simulink model "A2_NDI_AttitudeDynamics"  (R2017b)
settings: Solver=VariableStepAuto  StartTime=0.0  StopTime=300  FixedStep=1  MaxStep=0.1  RelTol=1e-6  EnableMultiTasking=on
StopFcn:
  | attitudePlot = animateAttitude(rotmOut, 0.016);
  | attitudePlot.plotInit;
values from neighbouring files (symbols this model uses):
  J_sat = [2.5 2.5 2.5]    [AttitudeDynamicsData.m]
  T_disturb = ones(1,3) * 0.1E-3    [AttitudeDynamicsData.m]
libraries: SatelliteLibrary x11, simulink x1
settings Model: Creator=Huib  LastModifiedBy=Huib
settings DataIOCC: LimitDataPoints=on
settings OptimizationCC: LifeSpan=inf
settings DebuggingCC: AllowSymbolicDim=off  SFUnexpectedBacktrackingDiag=warning  SFNoUnconditionalDefaultTransitionDiag=warning  SFExecutionAtInitializationDiag=none
settings ModelReferenceCC: PropagateSignalLabelsOutOfModel=off
settings CodeAppCC: StateflowObjectComments=on
settings GRTTargetCC: TargetLangStandard=C89/C90 (ANSI)
settings ConfigComp: CovMetricSettings=dw  CovHtmlReporting=on  CovSaveCumulativeToWorkspaceVar=on  CovSaveSingleToWorkspaceVar=on  CovExternalEMLEnable=off

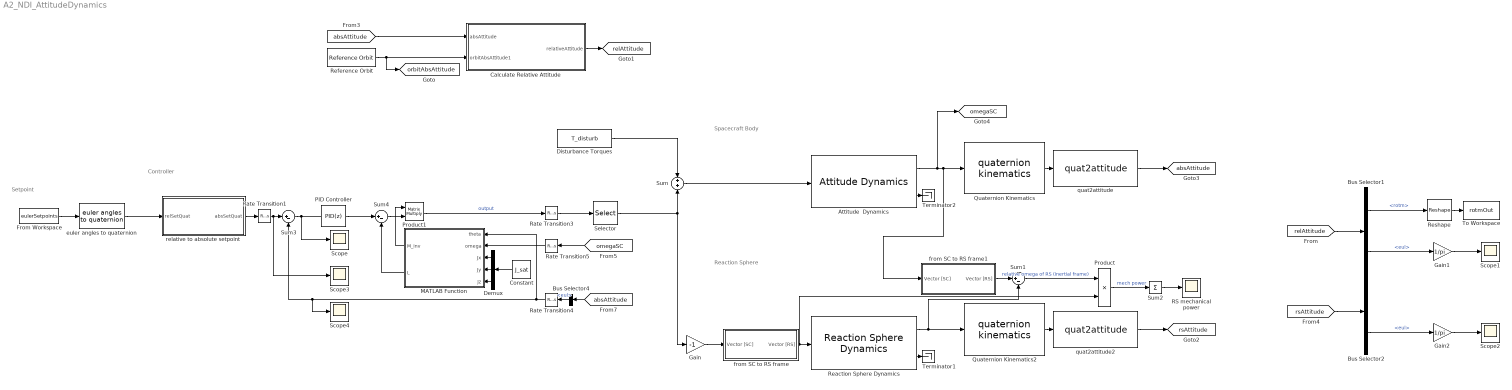
== system A2_NDI_AttitudeDynamics ==
  note: Setpoint
  note: Reaction Sphere
  note: Controller
  note: Spacecraft Body
  Attitude  Dynamics : SatelliteLibrary/Attitude Dynamics  J11=J_sat(1)  J22=J_sat(2)  J33=J_sat(3)  omega0=w_zero
  Bus Selector1 : BusSelector  OutputSignals=rotm,eul
  Bus Selector2 : BusSelector  OutputSignals=rotm,eul
  Bus Selector4 : BusSelector  OutputSignals=eul
  Calculate Relative Attitude : Subsystem
  Constant : Constant  Value=J_sat
  Demux : Demux  Outputs=3
  Disturbance Torques : Constant  Value=T_disturb
  From Workspace : FromWorkspace  VariableName=eulerSetpoints  SampleTime=0  Interpolate=off  OutputAfterFinalValue=Holding final value
  Gain : Gain  Gain=-1
  Gain1 : Gain  Gain=1/pi
  Gain2 : Gain  Gain=1/pi
  MATLAB Function : MATLAB Function  TreatAsAtomicUnit=on
  PID Controller : simulink/Continuous/PID Controller  Controller=PID  TimeDomain=Discrete-time  SampleTime=-1  IntegratorMethod=Forward Euler  FilterMethod=Forward Euler  Form=Parallel  UseFilter=off  ControllerParametersSource=internal  P=0.086943  I=0.001563  D=0.9084  N=100  InitialConditionSource=internal  InitialConditionForIntegrator=0  InitialConditionForFilter=0  ExternalReset=none  LimitOutput=off  UpperSaturationLimit=inf  LowerSaturationLimit=-inf  LinearizeAsGain=on  AntiWindupMode=none  Kb=1  TrackingMode=off  Kt=1  PParamMin=[]  PParamMax=[]  IParamMin=[]  IParamMax=[]  DParamMin=[]  DParamMax=[]  NParamMin=[]  NParamMax=[]  KbParamMin=[]  KbParamMax=[]  KtParamMin=[]  KtParamMax=[]  POutMin=[]  POutMax=[]  IOutMin=[]  IOutMax=[]  DOutMin=[]  DOutMax=[]  NOutMin=[]  NOutMax=[]  KbOutMin=[]  KbOutMax=[]  KtOutMin=[]  KtOutMax=[]  IntegratorOutMin=[]  IntegratorOutMax=[]  FilterOutMin=[]  FilterOutMax=[]  SumOutMin=[]  SumOutMax=[]  SumI1OutMin=[]  SumI1OutMax=[]  SumI2OutMin=[]  SumI2OutMax=[]  SumI3OutMin=[]  SumI3OutMax=[]  SumDOutMin=[]  SumDOutMax=[]  SaturationOutMin=[]  SaturationOutMax=[]  IntegratorContinuousStateAttributes=''  IntegratorStateMustResolveToSignalObject=off  IntegratorRTWStateStorageClass=Auto  FilterContinuousStateAttributes=''  FilterStateMustResolveToSignalObject=off  FilterRTWStateStorageClass=Auto  DifferentiatorICPrevScaledInput=0  DifferentiatorOutMin=[]  DifferentiatorOutMax=[]  InitialConditionSetting=State (most efficient)  FilterDiffOutCoefMin=[]  FilterDiffOutCoefMax=[]  SumDenOutMin=[]  SumDenOutMax=[]  SumNumOutMin=[]  SumNumOutMax=[]  ReciprocalOutMin=[]  ReciprocalOutMax=[]  DivideOutMin=[]  DivideOutMax=[]  TunerSelectOption=Transfer Function Based (PID Tuner App)
  Product : Product
  Product1 : Product  Multiplication=Matrix(*)
  Quaternion Kinematics : SatelliteLibrary/quaternion kinematics  q_0=q_zero
  Quaternion Kinematics2 : SatelliteLibrary/quaternion kinematics  q_0=q_zero
  RS mechanical power : Scope
  Rate Transition1 : RateTransition  OutPortSampleTime=0.1
  Rate Transition3 : RateTransition
  Rate Transition4 : RateTransition  OutPortSampleTime=0.1
  Rate Transition5 : RateTransition  OutPortSampleTime=0.1
  Reaction Sphere Dynamics : SatelliteLibrary/Reaction Sphere Dynamics  J=0.005567928416632  omega0=[0 0 0]
  Reference Orbit : SatelliteLibrary/Reference Orbit  orbitAltitude=700  gravParam=398600.4418  planetRadius=6371
  Reshape : Reshape  OutputDimensions=[9,1]
  Scope{,1..4} (5 alike) : Scope
  Selector : Selector  InputPortWidth=3  IndexOptions=Index vector (dialog)  Indices=[3 2 1]  OutputSizes=1
  Sum : Sum  Inputs=+|+
  Sum1 : Sum  Inputs=|+-
  Sum2 : Sum  Inputs=+
  Sum3 : Sum  Inputs=|+-
  Sum4 : Sum  Inputs=|+-
  Terminator1 : Terminator
  Terminator2 : Terminator
  To Workspace : ToWorkspace  VariableName=rotmOut  SaveFormat=Timeseries  SampleTime=-1
  euler angles to quaternion : SatelliteLibrary/euler angles to quaternion
  from SC to RS frame : Subsystem
  from SC to RS frame1 : Subsystem
  quat2attitude : SatelliteLibrary/quat2attitude
  quat2attitude2 : SatelliteLibrary/quat2attitude
  relative to absolute setpoint : Subsystem
  tag scope: absAttitude=global, omegaSC=global, orbitAbsAttitude=global, relAttitude=global, rsAttitude=global
  wires:
  Attitude  Dynamics/1 -> [omegaSC], from SC to RS frame1/1(Vector [SC]), Quaternion Kinematics/1
  Quaternion Kinematics/1 -> quat2attitude/1
  Sum/1 -> Attitude  Dynamics/1
  Reshape/1 -> To Workspace/1
  Bus Selector1/1 -> Reshape/1  "<rotm>"
  Gain1/1 -> Scope1/1
  Sum1/1 -> Product/1  "relative omega of RS (inertial frame)"
  Product/1 -> Sum2/1  "mech power"
  Bus Selector1/2 -> Gain1/1  "<eul>"
  [absAttitude] -> Calculate Relative Attitude/1(absAttitude)
  Calculate Relative Attitude/1(relativeAttitude) -> [relAttitude]
  quat2attitude/1 -> [absAttitude]
  Reference Orbit/1 -> [orbitAbsAttitude], Calculate Relative Attitude/2(orbitAbsAttitude1)
  Disturbance Torques/1 -> Sum/1
  [relAttitude] -> Bus Selector1/1
  From Workspace/1 -> euler angles to quaternion/1
  [rsAttitude] -> Bus Selector2/1
  Reaction Sphere Dynamics/1 -> Sum1/2, Quaternion Kinematics2/1
  Quaternion Kinematics2/1 -> quat2attitude2/1
  quat2attitude2/1 -> [rsAttitude]
  Gain/1 -> from SC to RS frame/1(Vector [SC])
  from SC to RS frame1/1(Vector [RS]) -> Sum1/1
  from SC to RS frame/1(Vector [RS]) -> Product/2, Reaction Sphere Dynamics/1
  Reaction Sphere Dynamics/2 -> Terminator1/1
  Attitude  Dynamics/2 -> Terminator2/1
  Bus Selector2/2 -> Gain2/1  "<eul>"
  Gain2/1 -> Scope2/1
  Sum2/1 -> RS mechanical power/1
  Demux/1 -> MATLAB Function/3(Jx)
  Demux/2 -> MATLAB Function/4(Jy)
  Demux/3 -> MATLAB Function/5(Jz)
  Constant/1 -> Demux/1
  [omegaSC] -> Rate Transition5/1
  Bus Selector4/1 -> Rate Transition4/1  "<eul>"
  [absAttitude] -> Bus Selector4/1
  Sum4/1 -> Product1/2
  MATLAB Function/1(M_inv) -> Product1/1
  MATLAB Function/2(L) -> Sum4/2
  Product1/1 -> Rate Transition3/1  "output"
  Sum3/1 -> PID Controller/1, Scope/1
  PID Controller/1 -> Sum4/1
  Rate Transition3/1 -> Selector/1
  Rate Transition1/1 -> Scope3/1, Sum3/1
  Rate Transition4/1 -> MATLAB Function/1(theta), Scope4/1, Sum3/2
  Rate Transition5/1 -> MATLAB Function/2(omega)
  Selector/1 -> Gain/1, Sum/2
  euler angles to quaternion/1 -> relative to absolute setpoint/1(relSetQuat)
  relative to absolute setpoint/1(absSetQuat) -> Rate Transition1/1

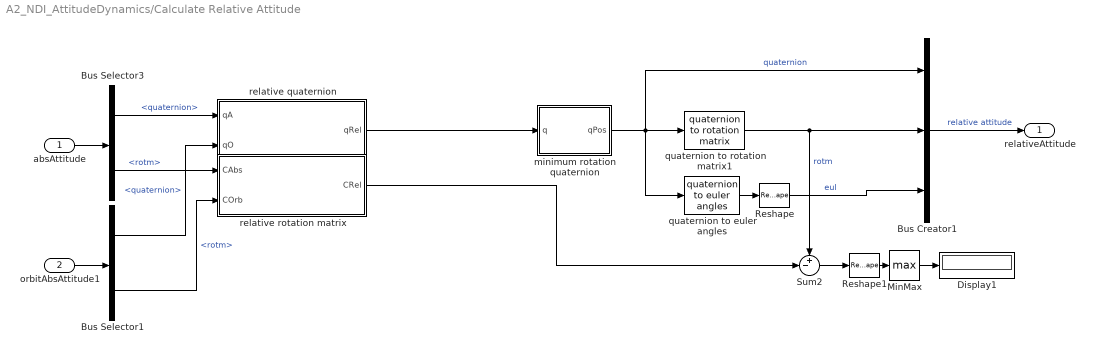
== system A2_NDI_AttitudeDynamics/Calculate Relative Attitude ==
  absAttitude : Inport
  orbitAbsAttitude1 : Inport  Port=2
  Bus Creator1 : BusCreator  Inputs=3
  Bus Selector1 : BusSelector  OutputSignals=quaternion,rotm
  Bus Selector3 : BusSelector  OutputSignals=quaternion,rotm
  Display1 : Display
  MinMax : MinMax  Function=max  ZeroCross=off
  Reshape : Reshape
  Reshape1 : Reshape
  Sum2 : Sum  Inputs=+-|
  minimum rotation quaternion : MATLAB Function  TreatAsAtomicUnit=on
  quaternion to euler angles : SatelliteLibrary/quaternion to euler angles
  quaternion to rotation matrix1 : SatelliteLibrary/quaternion to rotation matrix
  relative quaternion : MATLAB Function  TreatAsAtomicUnit=on
  relative rotation matrix : MATLAB Function  TreatAsAtomicUnit=on
  relativeAttitude : Outport
  wires:
  Bus Selector1/1 -> relative quaternion/2(qO)  "<quaternion>"
  Bus Selector3/2 -> relative rotation matrix/1(CAbs)  "<rotm>"
  Reshape1/1 -> MinMax/1
  MinMax/1 -> Display1/1
  relative rotation matrix/1(CRel) -> Sum2/2
  quaternion to rotation matrix1/1 -> Sum2/1, Bus Creator1/2  "rotm"
  Bus Creator1/1 -> relativeAttitude/1  "relative attitude"
  minimum rotation quaternion/1(qPos) -> Bus Creator1/1, quaternion to euler angles/1, quaternion to rotation matrix1/1  "quaternion"
  quaternion to euler angles/1 -> Reshape/1
  Bus Selector3/1 -> relative quaternion/1(qA)  "<quaternion>"
  Sum2/1 -> Reshape1/1
  relative quaternion/1(qRel) -> minimum rotation quaternion/1(q)
  Bus Selector1/2 -> relative rotation matrix/2(COrb)  "<rotm>"
  absAttitude/1 -> Bus Selector3/1
  orbitAbsAttitude1/1 -> Bus Selector1/1
  Reshape/1 -> Bus Creator1/3  "eul"

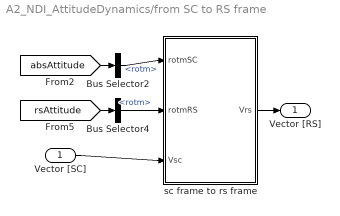
== system A2_NDI_AttitudeDynamics/from SC to RS frame ==
  Vector [SC] : Inport
  Bus Selector2 : BusSelector  OutputSignals=rotm
  Bus Selector4 : BusSelector  OutputSignals=rotm
  sc frame to rs frame : MATLAB Function  TreatAsAtomicUnit=on
  Vector [RS] : Outport
  wires:
  Vector [SC]/1 -> sc frame to rs frame/3(Vsc)
  sc frame to rs frame/1(Vrs) -> Vector [RS]/1
  [rsAttitude] -> Bus Selector4/1
  Bus Selector4/1 -> sc frame to rs frame/2(rotmRS)  "<rotm>"
  [absAttitude] -> Bus Selector2/1
  Bus Selector2/1 -> sc frame to rs frame/1(rotmSC)  "<rotm>"

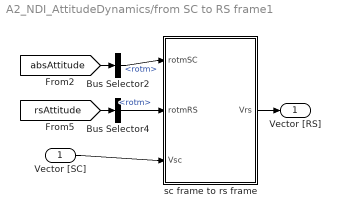
== system A2_NDI_AttitudeDynamics/from SC to RS frame1 ==
  Vector [SC] : Inport
  Bus Selector2 : BusSelector  OutputSignals=rotm
  Bus Selector4 : BusSelector  OutputSignals=rotm
  sc frame to rs frame : MATLAB Function  TreatAsAtomicUnit=on
  Vector [RS] : Outport
  wires:
  Vector [SC]/1 -> sc frame to rs frame/3(Vsc)
  sc frame to rs frame/1(Vrs) -> Vector [RS]/1
  [rsAttitude] -> Bus Selector4/1
  Bus Selector4/1 -> sc frame to rs frame/2(rotmRS)  "<rotm>"
  [absAttitude] -> Bus Selector2/1
  Bus Selector2/1 -> sc frame to rs frame/1(rotmSC)  "<rotm>"

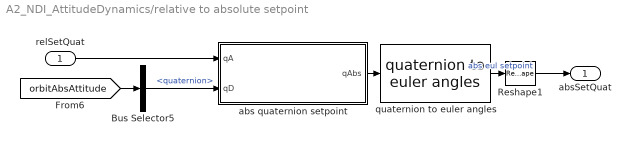
== system A2_NDI_AttitudeDynamics/relative to absolute setpoint ==
  relSetQuat : Inport
  Bus Selector5 : BusSelector  OutputSignals=quaternion
  Reshape1 : Reshape
  abs quaternion setpoint : MATLAB Function  TreatAsAtomicUnit=on
  quaternion to euler angles : SatelliteLibrary/quaternion to euler angles
  absSetQuat : Outport
  wires:
  abs quaternion setpoint/1(qAbs) -> quaternion to euler angles/1
  quaternion to euler angles/1 -> Reshape1/1  "abs eul setpoint"
  Reshape1/1 -> absSetQuat/1
  relSetQuat/1 -> abs quaternion setpoint/1(qA)
  Bus Selector5/1 -> abs quaternion setpoint/2(qD)  "<quaternion>"
  [orbitAbsAttitude] -> Bus Selector5/1

== matlab function A2_NDI_AttitudeDynamics/Calculate Relative Attitude/minimum rotation quaternion ==
  data: q input; qPos output
function qPos = minRotation(q)
    % converts quaternion to form of smalest angle (last element always <0, 1] )
    if q(4) < 0
        qPos = -q;
    else
        qPos = q;
    end
end

== matlab function A2_NDI_AttitudeDynamics/from SC to RS frame/sc frame to rs frame ==
  data: rotmSC input; Vrs output; rotmRS input; Vsc input
function ...
    Vrs               ...
  = sc2rs(            ...
    rotmSC,         ...
    rotmRS,         ...
    Vsc             ...
    )
    % transform vector in spacecraft (SC) frame into vector in
    % reactionsphere (RS) frame.
    Vrs = rotmRS' * rotmSC * Vsc;

end

== matlab function A2_NDI_AttitudeDynamics/Calculate Relative Attitude/relative rotation matrix ==
  data: CAbs input; COrb input; CRel output
function CRel = rotmatRelative(...
    CAbs, ... absolute rotation matrix orientation (in inertial reference frame)
    COrb  ... orbital frame rotation matrix orientation
    )

CRel = COrb' * CAbs;
end

== matlab function A2_NDI_AttitudeDynamics/Calculate Relative Attitude/relative quaternion ==
  data: qA input; qO input; qRel output
function qRel = quatRelative(...
    qA, ... absolute quaternion orientation (in inertial reference frame)
    qO  ... orbital frame quaternion orientation
    )
% Calculate the error quaternion
% q_... are standard quaternions with the vector part at the start

qOinv = [-qO(1:3); qO(4)];
qAmatrix = [ qA(4)  qA(3) -qA(2)  qA(1);...
            -qA(3)  qA(4)  qA(1)  qA(2);...
             qA(2) -qA(1)  qA(4)  qA(3);...
            -qA(1) -qA(2) -qA(3)  qA(4)];
qRel = qAmatrix * qOinv;
end

== matlab function A2_NDI_AttitudeDynamics/from SC to RS frame1/sc frame to rs frame ==
  data: rotmSC input; Vrs output; rotmRS input; Vsc input
function ...
    Vrs               ...
  = sc2rs(            ...
    rotmSC,         ...
    rotmRS,         ...
    Vsc             ...
    )
    % transform vector in spacecraft (SC) frame into vector in
    % reactionsphere (RS) frame.
    Vrs = rotmRS' * rotmSC * Vsc;

end

== matlab function A2_NDI_AttitudeDynamics/MATLAB Function ==
  data: theta input; M_inv output; omega input; Jx input; Jy input; Jz input; L output
function [M_inv, L] = fcn(theta, omega, Jx, Jy, Jz)
t1 = theta(1);
t2 = theta(2);
t3 = theta(3);
w1 = omega(1);
w2 = omega(2);
w3 = omega(3);

N_theta = [...
    1, sin(t1) * tan(t2), cos(t1) * tan(t2);...
    0,           cos(t1),         - sin(t1);...
    0, sin(t1) / cos(t2), cos(t1) / cos(t2)];

ddx_N_theta_omega = [...
      (cos(t2) * w2 - sin(t1) * w3)*tan(t2),         (sin(t1) * w2 + cos(t1)*w3) / cos(t2)^2, 0, 1, sin(t1) * tan(t2), cos(t1) * tan(t2);...
                - sin(t1) * w2 - cos(t1)*w3,                                               0, 0, 0,           cos(t1),         - sin(t1);...
    (cos(t1) * w2 - sin(t1) * w3) / cos(t2), (sin(t1) * w2 + cos(t1)*w3) * tan(t2) / cos(t2), 0, 0, sin(t1) / cos(t2), cos(t1) / cos(t2)];

J     = [Jx,  0,  0;...
          0, Jy,  0;...
          0,  0, Jz];

J_inv = [1/Jx,    0,     0;...
            0, 1/Jy,     0;...
            0,    0, 1/Jz];

Omega = [  0, -w3,  w2;...
          w3,   0, -w1;...
         -w2,  w1,   0];
        
M = ddx_N_theta_omega * [zeros(3,3); J_inv];

% dynamic inversion matrices
L = ddx_N_theta_omega * [N_theta*omega; -J_inv * Omega * J * omega];
M_inv = inv(M);

== matlab function A2_NDI_AttitudeDynamics/relative to absolute setpoint/abs quaternion setpoint ==
  data: qA input; qD input; qAbs output
function qAbs = quatAbsolute(...
    qA, ... relative quaternion orientation (in nadir pointing frame)
    qD  ... orbital frame quaternion orientation
    )
qD = [qD(1); qD(2); qD(3); qD(4)];
% q_... are standard quaternions with the vector part at the start
qAmatrix = [ qA(4)  qA(3) -qA(2)  qA(1);...
            -qA(3)  qA(4)  qA(1)  qA(2);...
             qA(2) -qA(1)  qA(4)  qA(3);...
            -qA(1) -qA(2) -qA(3)  qA(4)];
qAbs = qAmatrix * qD;

% converts quaternion to form of smalest angle (last element always <0, 1] )
end
